simulink model "sisotool_model"  (R2016b)
settings: Solver=VariableStepAuto  StartTime=0.0  StopTime=10.0  RelTol=1e-3
values from neighbouring files (symbols this model uses):
  den = [1 1021 4845]    [PI_control_design_of_DC_motor.m]
  KD = 0    [PI_control_design_of_DC_motor.m]
  KI = 0.28041*6.036    (= 1.69255476)    [PI_control_design_of_DC_motor.m]
  KP = 0.28041    [PI_control_design_of_DC_motor.m]
  num = [46163]    [PI_control_design_of_DC_motor.m]
settings Model: Creator=Christopher  LastModifiedBy=Christopher

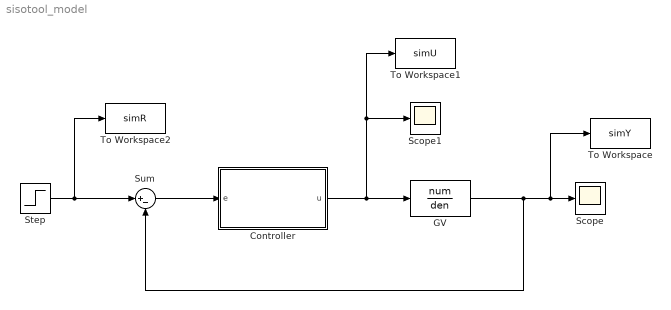
== system sisotool_model ==
  Controller : Subsystem
  GV : TransferFcn  Numerator=num  Denominator=den
  Scope : Scope
  Scope1 : Scope
  Step : Step  Time=5  Before=20  After=40  SampleTime=0
  Sum : Sum  Inputs=|+-
  To Workspace : ToWorkspace  VariableName=simY  SaveFormat=Structure With Time  SampleTime=-1
  To Workspace1 : ToWorkspace  VariableName=simU  SaveFormat=Structure With Time  SampleTime=-1
  To Workspace2 : ToWorkspace  VariableName=simR  SaveFormat=Structure With Time  SampleTime=-1
  wires:
  Controller/1(u) -> Scope1/1, To Workspace1/1, GV/1
  Step/1 -> To Workspace2/1, Sum/1
  Sum/1 -> Controller/1(e)
  GV/1 -> Sum/2, To Workspace/1, Scope/1

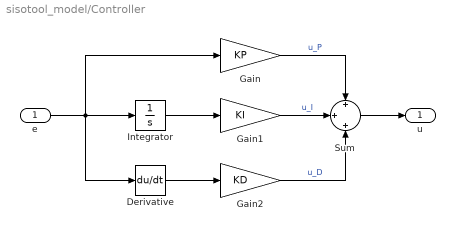
== system sisotool_model/Controller ==
  e : Inport
  Derivative : Derivative
  Gain : Gain  Gain=KP
  Gain1 : Gain  Gain=KI
  Gain2 : Gain  Gain=KD
  Integrator : Integrator
  Sum : Sum  Inputs=+|+|+
  u : Outport
  wires:
  Gain2/1 -> Sum/3  "u_D"
  Derivative/1 -> Gain2/1
  Gain1/1 -> Sum/2  "u_I"
  Sum/1 -> u/1
  Integrator/1 -> Gain1/1
  Gain/1 -> Sum/1  "u_P"
  e/1 -> Gain/1, Derivative/1, Integrator/1
